simulink model "HyEQsimulator_contr_Vdot0lines_w_hysteresis"  (Simulink 7.9)
settings: Solver=ode45  StartTime=0.0  StopTime=T  MaxStep=MaxStep  RelTol=RelTol
values from neighbouring files (symbols this model uses):
  C = 0.1    [initialization.m]
  Ides = Vdes^2/(E*R)    (= 3.26666666667)    [initialization.m]
  J = 1e8    (= 100000000)    [initialization.m]
  K0 = 0    [initialization.m]
  K1 = 0    [initialization.m]
  L = 0.2    [initialization.m]
  R = 3    [initialization.m]
  rule = 1    [initialization.m]
  T = 15    [initialization.m]
  Vdes = 7    [initialization.m]
  x0 = [0 5 5 1]    [converter10_1.mat]    (also in converter10_2.mat = [4 3 5 1]; converter10_3.mat = [6 2 5 1]; converter10_4.mat = [8 3 5 1]; converter10_5.mat = [5 0 5 1])
libraries: simulink x3
settings Model: Creator=s070289  LastModifiedBy=s070289

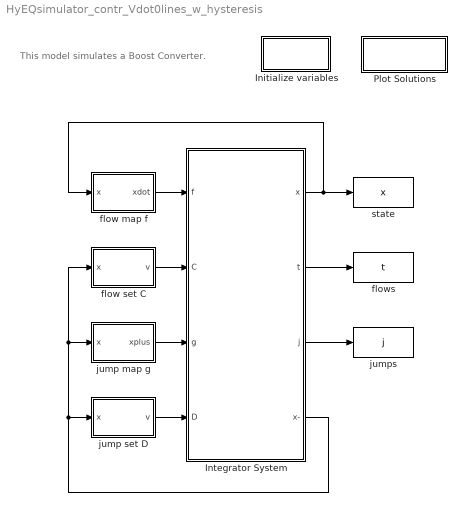
== system HyEQsimulator_contr_Vdot0lines_w_hysteresis ==
  note: This model simulates a Boost Converter.
  Initialize variables : Subsystem
      settings: OpenFcn=initialization
      mask Display: disp('Double Click\n to Initialize')
  Integrator System : Subsystem  mask(Hybrid Integrator){T=T, J=J, x0=x0}
      mask prompts: T "Flow Horizon"; J "Jump Horizon"; x0 "Initial Condition"
      mask help:
      | This block integrates the state of the hybrid system defined by the flow map f (first input), the flow set C (second input), the jump map g (third input) and the jump set D (fourth input).
      | Starting from the initial condition x0 (last mask parameter), the system's state x evolves continuously within the set C, according to f(x,u), but is also subject to jumps within D, according to g(x,u).
      | The block also stops the simulation when the time t is greater than the flow horizon T (first mask parameter), or when the number of jumps j is greater than the jump horizon J (second mask parameter).
      | The outputs of the blocks are respectively x(t), t, j, x(t-).
      mask Help:
      | This block integrates the state of the hybrid system defined by the flow map f (first input), the flow set C (second input), the jump map g (third input) and the jump set D (fourth input).
      | <br>
      | Starting from the initial condition x0 (last mask parameter), the system's state x evolves continuously within the set C, according to f(x,u), but is also subject to jumps within D, according to g(x,u).
      | <br>
      | The block also stops the simulation when the time t is greater than the flow horizon T (first mask parameter), or when the number of jumps j is greater than the jump horizon J (second mask parameter).
      | <br>
      | The outputs of the blocks are respectively x(t), t, j, x(t-).
      | <br>
      | You can right click on the block and "Look under mask" to see what's inside the block.
      | Finally, refer to the manual (HybridSimulator_vXX.pdf) for more detailed information on how this hybrid simulator works.
  Plot Solutions : Subsystem
      settings: OpenFcn=postprocessing
      mask Display: disp('Double Click to\n Plot Solutions')
  flow map f : MATLAB Function  TreatAsAtomicUnit=on
  flow set C : MATLAB Function  TreatAsAtomicUnit=on
  flows : ToWorkspace  VariableName=t  SampleTime=-1
  jump map g : MATLAB Function  TreatAsAtomicUnit=on
  jump set D : MATLAB Function  TreatAsAtomicUnit=on
  jumps : ToWorkspace  VariableName=j  SampleTime=-1
  state : ToWorkspace  VariableName=x  SampleTime=-1
  wires:
  flow map f/1(xdot) -> Integrator System/1(f)
  Integrator System/4(x-) -> jump map g/1(x), flow set C/1(x), jump set D/1(x)
  Integrator System/1(x) -> state/1, flow map f/1(x)
  flow set C/1(v) -> Integrator System/2(C)
  Integrator System/2(t) -> flows/1
  Integrator System/3(j) -> jumps/1
  jump set D/1(v) -> Integrator System/4(D)
  jump map g/1(xplus) -> Integrator System/3(g)

== system HyEQsimulator_contr_Vdot0lines_w_hysteresis/Initialize variables ==

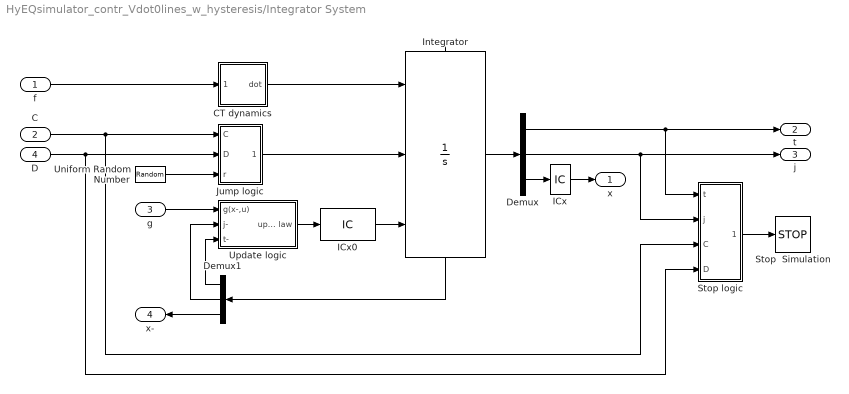
== system HyEQsimulator_contr_Vdot0lines_w_hysteresis/Integrator System ==
  f : Inport
  C : Inport  Port=2
  g : Inport  Port=3
  D : Inport  Port=4
  CT dynamics : Subsystem
  Demux : Demux  Outputs=[1 1 -1]
  Demux1 : Demux  Outputs=[1 1 -1]
  ICx : InitialCondition  Value=x0
  ICx0 : InitialCondition  Value=[0; 0; x0(:)]
  Integrator : Integrator  ExternalReset=level hold  InitialConditionSource=external  ShowStatePort=on  ZeroCross=off
  Jump logic : Subsystem
  Stop  Simulation : Stop
  Stop logic : Subsystem
  Uniform Random Number : UniformRandomNumber  Minimum=0  Seed=abs(floor(100*rand))  SampleTime=0
  Update logic : Subsystem
  x : Outport
  t : Outport  Port=2
  j : Outport  Port=3
  x- : Outport  Port=4
  wires:
  Demux1/2 -> Update logic/2(j-)
  Demux1/1 -> Update logic/3(t-)
  g/1 -> Update logic/1(g(x-,u))
  Uniform Random Number/1 -> Jump logic/3(r)
  Jump logic/1(jump) -> Integrator/2
  Demux1/3 -> x-/1
  f/1 -> CT dynamics/1(f(x,u))
  D/1 -> Jump logic/2(D), Stop logic/4(D)
  C/1 -> Jump logic/1(C), Stop logic/3(C)
  Integrator/1 -> Demux/1
  Stop logic/1(stop) -> Stop  Simulation/1
  CT dynamics/1(dot) -> Integrator/1
  Update logic/1(update law) -> ICx0/1
  Demux/1 -> Stop logic/1(t), t/1
  Demux/2 -> Stop logic/2(j), j/1
  Integrator/State -> Demux1/1
  Demux/3 -> ICx/1
  ICx/1 -> x/1
  ICx0/1 -> Integrator/3

== system HyEQsimulator_contr_Vdot0lines_w_hysteresis/Plot Solutions ==

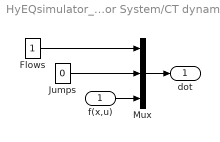
== system HyEQsimulator_contr_Vdot0lines_w_hysteresis/Integrator System/CT dynamics ==
  f(x,u) : Inport
  Flows : Constant
  Jumps : Constant  Value=0
  Mux : Mux  Inputs=[1 1 -1]
  dot : Outport
  wires:
  f(x,u)/1 -> Mux/3
  Mux/1 -> dot/1
  Flows/1 -> Mux/1
  Jumps/1 -> Mux/2

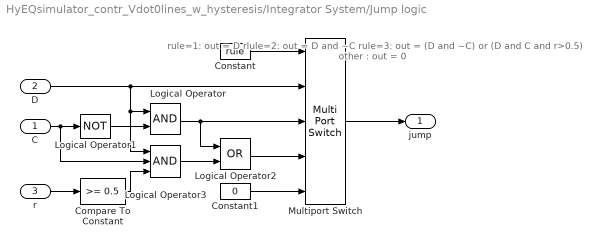
== system HyEQsimulator_contr_Vdot0lines_w_hysteresis/Integrator System/Jump logic ==
  note: rule=1:  out = D
      | rlule=2: out = D and ~C
      | rule=3:  out = (D and ~C)  or (D and C and r>0.5)
      | other :  out = 0
  C : Inport
  D : Inport  Port=2
  r : Inport  Port=3
  Compare To Constant : simulink/Logic and Bit Operations/Compare To Constant  relop=>=  const=0.5  OutDataTypeStr=uint8
  Constant : Constant  Value=rule
  Constant1 : Constant  Value=0
  Logical Operator : Logic  AllPortsSameDT=off  OutDataTypeStr=boolean
  Logical Operator1 : Logic  Operator=NOT  Inputs=1  AllPortsSameDT=off  OutDataTypeStr=boolean
  Logical Operator2 : Logic  Operator=OR  AllPortsSameDT=off  OutDataTypeStr=boolean
  Logical Operator3 : Logic  Inputs=3  AllPortsSameDT=off  OutDataTypeStr=boolean
  Multiport Switch : MultiPortSwitch  DataPortForDefault=Additional data port  zeroidx=off
  jump : Outport
  wires:
  Constant1/1 -> Multiport Switch/5
  Logical Operator3/1 -> Logical Operator2/2
  Compare To Constant/1 -> Logical Operator3/3
  Multiport Switch/1 -> jump/1
  Logical Operator2/1 -> Multiport Switch/4
  Logical Operator/1 -> Logical Operator2/1, Multiport Switch/3
  Logical Operator1/1 -> Logical Operator/2
  C/1 -> Logical Operator1/1, Logical Operator3/2
  r/1 -> Compare To Constant/1
  D/1 -> Multiport Switch/2, Logical Operator/1, Logical Operator3/1
  Constant/1 -> Multiport Switch/1

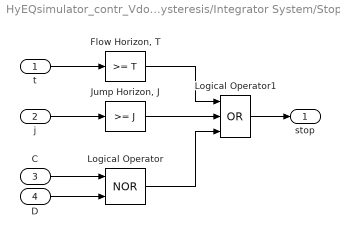
== system HyEQsimulator_contr_Vdot0lines_w_hysteresis/Integrator System/Stop logic ==
  t : Inport
  j : Inport  Port=2
  C : Inport  Port=3
  D : Inport  Port=4
  "Flow Horizon, T" : simulink/Logic and Bit Operations/Compare To Constant  relop=>=  const=T  OutDataTypeStr=uint8  ZeroCross=off
  "Jump Horizon, J" : simulink/Logic and Bit Operations/Compare To Constant  relop=>=  const=J  OutDataTypeStr=uint8  ZeroCross=off
  Logical Operator : Logic  Operator=NOR  AllPortsSameDT=off  OutDataTypeStr=boolean
  Logical Operator1 : Logic  Operator=OR  Inputs=3  AllPortsSameDT=off  OutDataTypeStr=boolean
  stop : Outport
  wires:
  Logical Operator1/1 -> stop/1
  C/1 -> Logical Operator/1
  j/1 -> "Jump Horizon, J"/1
  t/1 -> "Flow Horizon, T"/1
  D/1 -> Logical Operator/2
  Logical Operator/1 -> Logical Operator1/3
  "Jump Horizon, J"/1 -> Logical Operator1/2
  "Flow Horizon, T"/1 -> Logical Operator1/1

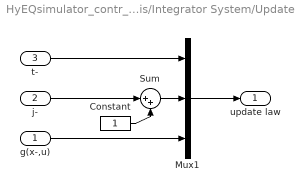
== system HyEQsimulator_contr_Vdot0lines_w_hysteresis/Integrator System/Update logic ==
  g(x-,u) : Inport
  j- : Inport  Port=2
  t- : Inport  Port=3
  Constant : Constant
  Mux1 : Mux  Inputs=[1 1 -1]
  Sum : Sum  Inputs=|++
  update law : Outport
  wires:
  Constant/1 -> Sum/2
  t-/1 -> Mux1/1
  g(x-,u)/1 -> Mux1/3
  j-/1 -> Sum/1
  Mux1/1 -> update law/1
  Sum/1 -> Mux1/2

== matlab function jump set D ==
  data: x input double; v output double; R parameter double; C parameter double; L parameter double; K0 parameter double; K1 parameter double; Vdes parameter double; Ides parameter double; eps parameter double
function v  = D(x, R, C, L, K0, K1, Vdes, Ides, eps) 

%%%%%%%%%%%%%%%%%%%%%%%%%%%%%%%%%%%%%%%%%%%%%%%%%%%%%%%%%%%%%%%%%%%%%%%%%%%
% Matlab Function  Author: Thomas A.F. Theunisse
%
% Project: Simulation of a hybrid system (Boost Converter)
%
% Name: D.m
%
% Description: Jump set for controller 2
%
% Version: 1.0
% Required files: - 
%%%%%%%%%%%%%%%%%%%%%%%%%%%%%%%%%%%%%%%%%%%%%%%%%%%%%%%%%%%%%%%%%%%%%%%%%%%

vC = x(1);
iL = x(2);
E = x(3);
q = round(x(4));

p11 = C/2;
p22 = L/2; 
A0 = -p11/(R*C);
B0 = p11*Vdes/(R*C)+p22*Ides/L;
C0 = -p11*Vdes/C+p22*E/L;
D0 = -p22*Ides*E/L;
A1 = -p11/(R*C);
B1 = p11*Vdes/(R*C);
C1 = p22*E/L;
D1 = -p22*Ides*E/L;

A0tilde = A0+K0*p11*Vdes/(R*C*E);
B0tilde = B0-K0*2*p11*Ides/C;
C0tilde = C0;
D0tilde = D0+K0*p22*Vdes*Ides/L;
A1tilde = A1+K1*p11*Vdes/(R*C*(Vdes-E));
B1tilde = B1+K1*2*p11*Vdes^2/(R*C*(E-Vdes));
C1tilde = C1;
D1tilde = D1+K1*p22*Vdes*Ides*E/(L*(Vdes-E));

gamma0 = A0tilde*vC.^2+B0tilde*vC+C0tilde*iL+D0tilde;
gamma1 = A1tilde*vC.^2+B1tilde*vC+C1tilde*iL+D1tilde;

%gamma0 = (vC-Vdes).*(-vC./R+iL) + (iL-Ides).*(-vC+E);
%gamma1 = -1/R*(vC-Vdes).*vC + E*(iL-Ides);

if ( q == 0 && gamma0 >= eps ) || ( q == 1 && gamma1 >= eps ) % jump condition
    v = 1;  % report jump
else
    v = 0;   % do not report jump
end

== matlab function flow map f ==
  data: x input double; xdot output double; R parameter int32; L parameter double; C parameter double
function xdot = f(x, R, L, C)

%%%%%%%%%%%%%%%%%%%%%%%%%%%%%%%%%%%%%%%%%%%%%%%%%%%%%%%%%%%%%%%%%%%%%%%%%%%
% Matlab Function  Author: Thomas A.F. Theunisse
%
% Project: Simulation of a hybrid system (Boost Converter)
%
% Name: f.m
%
% Description: Flow map
%
% Version: 1.0
% Required files: -
%%%%%%%%%%%%%%%%%%%%%%%%%%%%%%%%%%%%%%%%%%%%%%%%%%%%%%%%%%%%%%%%%%%%%%%%%%%

% flow map: xdot=f(x,u);
vC = x(1);
iL = x(2);
E = x(3);
q = round(x(4));

switch q
    case 0
        if vC <= E || iL >= 0;
            F = [-1/(R*C)*vC+1/C*iL; -1/L*vC+E/L];
        elseif vC > E && iL <= 0; 
            F = [-1/(R*C)*vC; 0];
        else
            F = [0; 0];
        end
    case 1
        F = [-1/(R*C)*vC; E/L];
    otherwise
        F = [0; 0];
%         disp('Warning on f: Unknown method.')
end
xdot = [F; 0; 0];

== matlab function flow set C ==
  data: x input double; v output double; R parameter double; C parameter double; L parameter double; K0 parameter double; K1 parameter double; Vdes parameter double; Ides parameter double; eps parameter double
function v  = C(x, R, C, L, K0, K1, Vdes, Ides, eps) 

%%%%%%%%%%%%%%%%%%%%%%%%%%%%%%%%%%%%%%%%%%%%%%%%%%%%%%%%%%%%%%%%%%%%%%%%%%%
% Matlab Function  Author: Thomas A.F. Theunisse
%
% Project: Simulation of a hybrid system (Boost Converter)
%
% Name: C.m
%
% Description: Flow set
%
% Version: 1.0
% Required files: - 
%%%%%%%%%%%%%%%%%%%%%%%%%%%%%%%%%%%%%%%%%%%%%%%%%%%%%%%%%%%%%%%%%%%%%%%%%%%

vC = x(1);
iL = x(2);
E = x(3);
q = round(x(4));

p11 = C/2;
p22 = L/2; 
A0 = -p11/(R*C);
B0 = p11*Vdes/(R*C)+p22*Ides/L;
C0 = -p11*Vdes/C+p22*E/L;
D0 = -p22*Ides*E/L;
A1 = -p11/(R*C);
B1 = p11*Vdes/(R*C);
C1 = p22*E/L;
D1 = -p22*Ides*E/L;

A0tilde = A0+K0*p11*Vdes/(R*C*E);
B0tilde = B0-K0*2*p11*Ides/C;
C0tilde = C0;
D0tilde = D0+K0*p22*Vdes*Ides/L;
A1tilde = A1+K1*p11*Vdes/(R*C*(Vdes-E));
B1tilde = B1+K1*2*p11*Vdes^2/(R*C*(E-Vdes));
C1tilde = C1;
D1tilde = D1+K1*p22*Vdes*Ides*E/(L*(Vdes-E));

gamma0 = A0tilde*vC.^2+B0tilde*vC+C0tilde*iL+D0tilde;
gamma1 = A1tilde*vC.^2+B1tilde*vC+C1tilde*iL+D1tilde;

%gamma0 = (vC-Vdes).*(-vC./R+iL) + (iL-Ides).*(-vC+E);
%gamma1 = -1/R*(vC-Vdes).*vC + E*(iL-Ides);

if ( q == 0 && gamma0 <= eps ) || ( q == 1 && gamma1 <= eps )  % flow condition
    v = 1;  % report flow
else
    v = 0;   % do not report flow
end

== matlab function jump map g ==
  data: x input double; xplus output double; R parameter double; C parameter double; L parameter double; K0 parameter double; K1 parameter double; Vdes parameter double; Ides parameter double; eps parameter double
function xplus = g(x, R, C, L, K0, K1, Vdes, Ides, eps)

%%%%%%%%%%%%%%%%%%%%%%%%%%%%%%%%%%%%%%%%%%%%%%%%%%%%%%%%%%%%%%%%%%%%%%%%%%%
% Matlab Function  Author: Thomas A.F. Theunisse
%
% Project: Simulation of a hybrid system (Boost Converter)
%
% Name: g.m
%
% Description: Jump map for controller 2
%
% Version: 1.0
% Required files: - 
%%%%%%%%%%%%%%%%%%%%%%%%%%%%%%%%%%%%%%%%%%%%%%%%%%%%%%%%%%%%%%%%%%%%%%%%%%%

vC = x(1);
iL = x(2);
E = x(3);
q = round(x(4));

p11 = C/2;
p22 = L/2; 
A0 = -p11/(R*C);
B0 = p11*Vdes/(R*C)+p22*Ides/L;
C0 = -p11*Vdes/C+p22*E/L;
D0 = -p22*Ides*E/L;
A1 = -p11/(R*C);
B1 = p11*Vdes/(R*C);
C1 = p22*E/L;
D1 = -p22*Ides*E/L;

A0tilde = A0+K0*p11*Vdes/(R*C*E);
B0tilde = B0-K0*2*p11*Ides/C;
C0tilde = C0;
D0tilde = D0+K0*p22*Vdes*Ides/L;
A1tilde = A1+K1*p11*Vdes/(R*C*(Vdes-E));
B1tilde = B1+K1*2*p11*Vdes^2/(R*C*(E-Vdes));
C1tilde = C1;
D1tilde = D1+K1*p22*Vdes*Ides*E/(L*(Vdes-E));

gamma0 = A0tilde*vC.^2+B0tilde*vC+C0tilde*iL+D0tilde;
gamma1 = A1tilde*vC.^2+B1tilde*vC+C1tilde*iL+D1tilde;

%gamma0 = (vC-Vdes).*(-vC./R+iL) + (iL-Ides).*(-vC+E);
%gamma1 = -1/R*(vC-Vdes).*vC + E*(iL-Ides);

% jump map

if q == 0 && gamma0 >= eps
    zplus = [vC; iL];
    qplus = 1;
elseif q == 1 && gamma1 >= eps
    zplus = [vC; iL];
    qplus = 0;    
else
    zplus = [vC; iL];
    qplus = q;    
end
    
xplus = [zplus; E; qplus];
